simulink library "turn_left_Gait"  (R2024a)
settings: Solver=VariableStepAuto  StartTime=0.0  StopTime=10.0  RelTol=1e-3
libraries: delay_and_stop_when_change x3, Plane_Movement_walk_right x2, Plane_Movement_walk_left x2
settings Model: Creator=renre  LastModifiedBy=leona

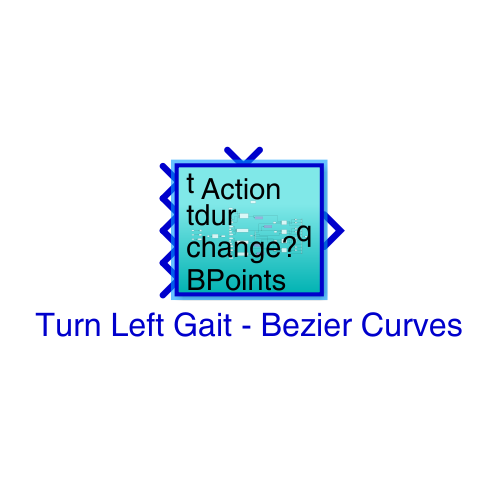
[thumbnail: Simulink's stored preview of the top-level diagram]
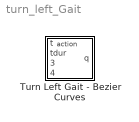
== system turn_left_Gait ==
  Turn Left Gait - Bezier Curves : Subsystem

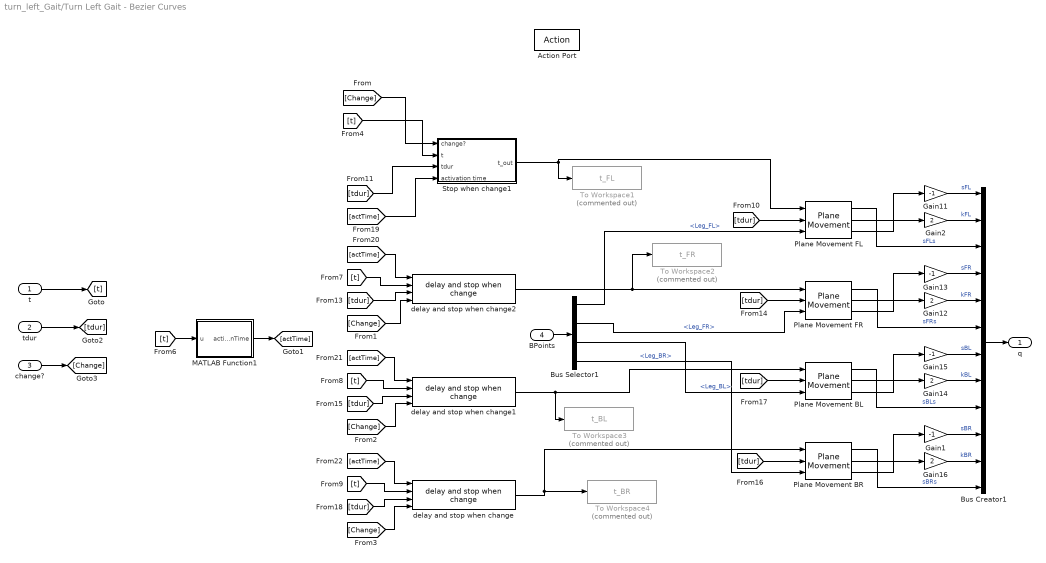
== system turn_left_Gait/Turn Left Gait - Bezier Curves ==
  t : Inport
  tdur : Inport  Port=2
  change? : Inport  Port=3
  BPoints : Inport  Port=4
  Action Port : ActionPort  InitializeStates=reset
  Bus Creator1 : BusCreator  Inputs=12
  Bus Selector1 : BusSelector  OutputSignals=Leg_FL,Leg_FR,Leg_BL,Leg_BR
  Gain{1,11,13,15} (4 alike) : Gain  Gain=-1
  Gain{2,12,14,16} (4 alike) : Gain  Gain=2
  MATLAB Function1 : MATLAB Function  TreatAsAtomicUnit=on
  Plane Movement BL : Plane_Movement_walk_right/Plane Movement  SystemSampleTime=-1  VariantActivationTime=update diagram  AllowFlexibleInterface=on  Latency=0  AutoFrameSizeCalculation=off
  Plane Movement BR : Plane_Movement_walk_right/Plane Movement  SystemSampleTime=-1  VariantActivationTime=update diagram  AllowFlexibleInterface=on  Latency=0  AutoFrameSizeCalculation=off
  Plane Movement FL : Plane_Movement_walk_left/Plane Movement  SystemSampleTime=-1  VariantActivationTime=update diagram  AllowFlexibleInterface=on  Latency=0  AutoFrameSizeCalculation=off
  Plane Movement FR : Plane_Movement_walk_left/Plane Movement  SystemSampleTime=-1  VariantActivationTime=update diagram  AllowFlexibleInterface=on  Latency=0  AutoFrameSizeCalculation=off
  Stop when change1 : Subsystem
  To Workspace1 : ToWorkspace  Commented=on  VariableName=t_FL  SaveFormat=Structure With Time  SampleTime=-1
  To Workspace2 : ToWorkspace  Commented=on  VariableName=t_FR  SaveFormat=Structure  SampleTime=-1
  To Workspace3 : ToWorkspace  Commented=on  VariableName=t_BL  SaveFormat=Structure  SampleTime=-1
  To Workspace4 : ToWorkspace  Commented=on  VariableName=t_BR  SaveFormat=Structure  SampleTime=-1
  delay and stop when change : delay_and_stop_when_change/delay and stop when change  delay=0.75
  delay and stop when change1 : delay_and_stop_when_change/delay and stop when change  delay=0.25
  delay and stop when change2 : delay_and_stop_when_change/delay and stop when change  delay=0.5
  q : Outport
  wires:
  [tdur] -> Plane Movement FL/2
  [tdur] -> delay and stop when change/3
  [actTime] -> delay and stop when change/1
  [tdur] -> Stop when change1/3(tdur)
  [tdur] -> delay and stop when change2/3
  [tdur] -> Plane Movement FR/2
  [Change] -> Stop when change1/1(change?)
  [tdur] -> Plane Movement BL/2
  Gain15/1 -> Bus Creator1/7  "sBL"
  Gain14/1 -> Bus Creator1/8  "kBL"
  change?/1 -> [Change]
  MATLAB Function1/1(activationTime) -> [actTime]
  [t] -> delay and stop when change/2
  [t] -> Stop when change1/2(t)
  [Change] -> delay and stop when change1/4
  [t] -> delay and stop when change1/2
  [t] -> MATLAB Function1/1(u)
  Bus Selector1/4 -> Plane Movement BR/3  "<Leg_BR>"
  Plane Movement BL/2 -> Gain14/1
  Bus Selector1/3 -> Plane Movement BL/3  "<Leg_BL>"
  delay and stop when change2/1 -> To Workspace2/1, Plane Movement FR/1
  Bus Selector1/1 -> Plane Movement FL/3  "<Leg_FL>"
  t/1 -> [t]
  Gain16/1 -> Bus Creator1/11  "kBR"
  BPoints/1 -> Bus Selector1/1
  Plane Movement FL/1 -> Bus Creator1/3  "sFLs"
  Plane Movement FR/1 -> Bus Creator1/6  "sFRs"
  [actTime] -> delay and stop when change2/1
  Gain2/1 -> Bus Creator1/2  "kFL"
  Gain1/1 -> Bus Creator1/10  "sBR"
  Plane Movement BL/1 -> Bus Creator1/9  "sBLs"
  [tdur] -> delay and stop when change1/3
  Gain11/1 -> Bus Creator1/1  "sFL"
  Stop when change1/1(t_out) -> Plane Movement FL/1, To Workspace1/1
  Gain12/1 -> Bus Creator1/5  "kFR"
  delay and stop when change1/1 -> To Workspace3/1, Plane Movement BL/1
  Bus Creator1/1 -> q/1
  [actTime] -> Stop when change1/4(activation time)
  delay and stop when change/1 -> To Workspace4/1, Plane Movement BR/1
  [Change] -> delay and stop when change/4
  Plane Movement FL/2 -> Gain2/1
  [Change] -> delay and stop when change2/4
  [t] -> delay and stop when change2/2
  Gain13/1 -> Bus Creator1/4  "sFR"
  Plane Movement BR/1 -> Bus Creator1/12  "sBRs"
  [actTime] -> delay and stop when change1/1
  Plane Movement BR/2 -> Gain16/1
  Bus Selector1/2 -> Plane Movement FR/3  "<Leg_FR>"
  tdur/1 -> [tdur]
  [tdur] -> Plane Movement BR/2
  Plane Movement FR/2 -> Gain12/1
  Plane Movement FL/3 -> Gain11/1
  Plane Movement FR/3 -> Gain13/1
  Plane Movement BL/3 -> Gain15/1
  Plane Movement BR/3 -> Gain1/1

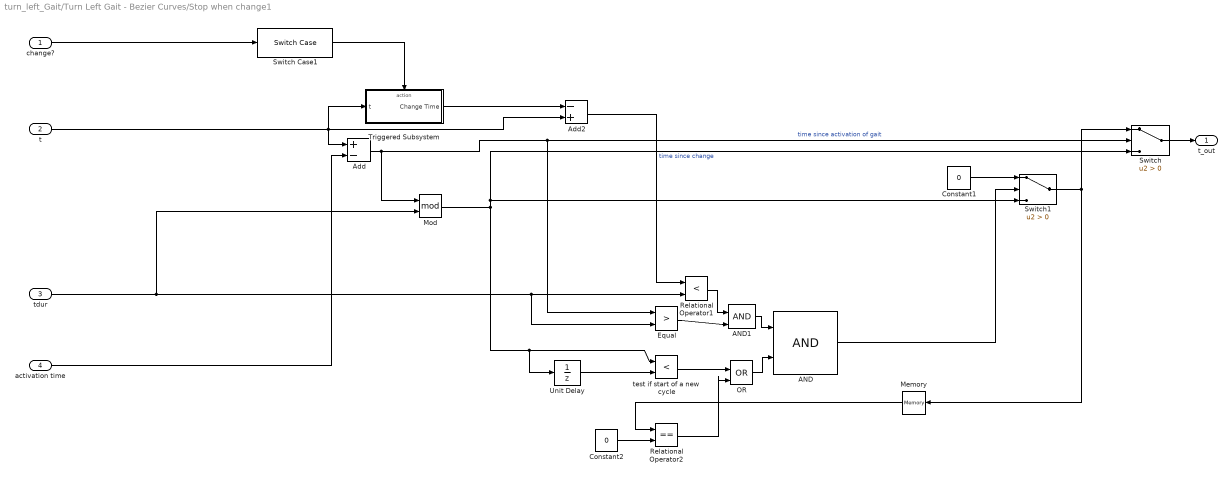
== system turn_left_Gait/Turn Left Gait - Bezier Curves/Stop when change1 ==
  change? : Inport
  t : Inport  Port=2
  tdur : Inport  Port=3
  activation time : Inport  Port=4
  AND : Logic  IconShape=distinctive  AllPortsSameDT=off  OutDataTypeStr=boolean
  AND1 : Logic  IconShape=distinctive  AllPortsSameDT=off  OutDataTypeStr=boolean
  Add : Sum  Inputs=+-
  Add2 : Sum  Inputs=-+
  Constant1 : Constant  Value=0
  Constant2 : Constant  Value=0
  Equal : RelationalOperator  Operator=>  OutDataTypeStr=boolean  RndMeth=Simplest  InputSameDT=off
  Memory : Memory
  Mod : Math  Operator=mod
  OR : Logic  Operator=OR  IconShape=distinctive  AllPortsSameDT=off  OutDataTypeStr=boolean
  Relational Operator1 : RelationalOperator  Operator=<  OutDataTypeStr=boolean  RndMeth=Simplest  InputSameDT=off
  Relational Operator2 : RelationalOperator  Operator===  OutDataTypeStr=boolean  RndMeth=Simplest  InputSameDT=off
  Switch : Switch  Criteria=u2 > Threshold  SaturateOnIntegerOverflow=off  InputSameDT=off
  Switch Case1 : SwitchCase  ShowDefaultCase=off
  Switch1 : Switch  Criteria=u2 > Threshold  SaturateOnIntegerOverflow=off  InputSameDT=off
  Triggered Subsystem : Subsystem  TreatAsAtomicUnit=on
  Unit Delay : UnitDelay  SampleTime=-1  HasFrameUpgradeWarning=on
  test if start of a new cycle : RelationalOperator  Operator=<  OutDataTypeStr=boolean  RndMeth=Simplest  InputSameDT=off
  t_out : Outport
  wires:
  Relational Operator1/1 -> AND1/1
  Switch Case1/1 -> Triggered Subsystem/Action
  AND1/1 -> AND/1
  Mod/1 -> test if start of a new cycle/1, Unit Delay/1, Switch1/3, Switch/3
  change?/1 -> Switch Case1/1
  Triggered Subsystem/1(Change Time) -> Add2/1
  tdur/1 -> Mod/2, Equal/2, Relational Operator1/2
  Unit Delay/1 -> test if start of a new cycle/2
  AND/1 -> Switch1/2
  Switch1/1 -> Switch/1, Memory/1
  Constant2/1 -> Relational Operator2/2
  Add2/1 -> Relational Operator1/1  "time since change"
  test if start of a new cycle/1 -> OR/1
  Memory/1 -> Relational Operator2/1
  Relational Operator2/1 -> OR/2
  Switch/1 -> t_out/1
  OR/1 -> AND/2
  Equal/1 -> AND1/2
  activation time/1 -> Add/2
  Add/1 -> Mod/1, Equal/1, Switch/2  "time since activation of gait"
  t/1 -> Triggered Subsystem/1(t), Add/1, Add2/2
  Constant1/1 -> Switch1/1

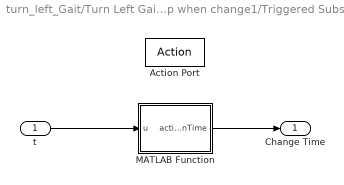
== system turn_left_Gait/Turn Left Gait - Bezier Curves/Stop when change1/Triggered Subsystem ==
  t : Inport
  Action Port : ActionPort  InitializeStates=reset  ActionPortLabel=case [ 1 ]:
  MATLAB Function : MATLAB Function  TreatAsAtomicUnit=on
  Change Time : Outport
  wires:
  t/1 -> MATLAB Function/1(u)
  MATLAB Function/1(activationTime) -> Change Time/1

== matlab function turn_left_Gait/Turn Left Gait - Bezier Curves/Stop when change1/Triggered Subsystem/MATLAB Function ==
  data: u input; activationTime output
function activationTime = getActivationTime(u)
    persistent t_start
    if isempty(t_start)
        t_start = u;
    end
    activationTime = t_start;
end

== matlab function turn_left_Gait/Turn Left Gait - Bezier Curves/MATLAB Function1 ==
  data: u input; activationTime output
function activationTime = getActivationTime(u)
    persistent t_start
    if isempty(t_start)
        t_start = u;
    end
    activationTime = t_start;
end
